simulink model "assembly_crl"  (R2022b)
settings: Solver=FixedStepDiscrete  StartTime=0.0  StopTime=5  RelTol=1e-3  EnableMultiTasking=on
InitFcn:
  | frameSize = 32;
  | numChannels = 2;
  | fs = 44100;
  | maxStages = 4;
  | stagesPerChannel = [1 1];
  | coeffs = [1 0  0 1 0 0; 1 0 0 1 0 0];
  | 
  | firCoeffs = single(zeros(1,32));
  | activeCoeffSet = [0 0];
undefined symbols (not defined in the file or in its folder): carModel, mode
libraries: FeaturePath x1
settings Model: Creator=ap71173  LastModifiedBy=kl13806
settings SolverCC: AlgebraicLoopSolver=TrustRegion
settings OptimizationCC: DefaultParameterBehavior=Inlined  DefaultUnderspecifiedDataType=single  MaxStackSize=2048  EfficientTunableParamExpr=on
settings DebuggingCC: InheritedTsInSrcMsg=none  MultiTaskDSMMsg=none  ParameterPrecisionLossMsg=none  ParameterTunabilityLossMsg=error  UnconnectedInputMsg=warning  UnconnectedOutputMsg=warning  UnconnectedLineMsg=warning  UnknownTsInhSupMsg=none  SFUnexpectedBacktrackingDiag=warning  SFNoUnconditionalDefaultTransitionDiag=warning  SFExecutionAtInitializationDiag=none  SFMachineParentedDataDiag=warning  ArithmeticOperatorsInVariantConditions=warning
settings HardwareCC: ProdBitPerPointer=32  ProdBitPerSizeT=32  ProdBitPerPtrDiffT=32  ProdLargestAtomicInteger=Long  ProdLargestAtomicFloat=Double  ProdEndianess=BigEndian  ProdWordSize=32  ProdHWDeviceType=Custom Processor->Custom  TargetBitPerPointer=64  TargetBitPerSizeT=64  TargetBitPerPtrDiffT=64  TargetLongLongMode=on  TargetIntDivRoundTo=Zero  TargetEndianess=LittleEndian  TargetWordSize=64  TargetHWDeviceType=MATLAB Host
settings ModelReferenceCC: EnableRefExpFcnMdlSchedulingChecks=on
settings SFSimCC: SimUseLocalCustomCode=off  MATLABDynamicMemAlloc=off  CustomCodeUndefinedFunction=UseInterfaceOnly
settings RTWCC: Description=Embedded Coder (host-based shared library target)  SystemTargetFile=ert_shrlib.tlc  TemplateMakefile=ert_default_tmf  GenerateReport=on  RetainRTWFile=on  RTWUseLocalCustomCode=off  Toolchain=ADSP-SC58x v2.3 | gmake makefile (64-bit Windows)  BuildConfiguration=Release - ADSP-SC584  IncludeHyperlinkInReport=on  LaunchReport=on  GenerateTraceInfo=on  GenerateTraceReport=on  GenerateTraceReportSl=on  GenerateTraceReportSf=on  GenerateTraceReportEml=on  GenerateCodeMetricsReport=on  GenerateCodeReplacementReport=on  DLArmComputeVersion=19.05
settings CodeAppCC: ForceParamTrailComments=on  IgnoreCustomStorageClasses=off  OperatorAnnotations=on  SimulinkDataObjDesc=on  SFDataObjDesc=on  MATLABFcnDesc=on  InsertBlockDesc=on  StateflowObjectComments=on  MATLABSourceComments=on
settings STFCustomTargetCC: TargetLangStandard=C99 (ISO)  CodeReplacementLibrary=SHARC+ code replacement libarary  MultiwordLength=256  ParMdlRefBuildCompliant=on  CompOptLevelCompliant=on  CombineOutputUpdateFcns=on  ERTCustomFileBanners=on  SupportContinuousTime=off  SupportNonInlinedSFcns=off  RemoveResetFunc=on  SupportVariableSizeSignals=on  MATLABClassNameForMDSCustomization=Simulink.SoftwareTarget.ERTCustomization  ModelStepFunctionPrototypeControlCompliant=on  UseToolchainInfoCompliant=on  SystemTargetFile=ert_shrlib.tlc
settings ERTTargetCC: TargetLangStandard=C99 (ISO)  CodeReplacementLibrary=SHARC+ code replacement libarary  ConcurrentExecutionCompliant=off  SupportVariableSizeSignals=on  CPPClassGenCompliant=off  InlinedParameterPlacement=NonHierarchical  ERTCustomFileTemplate=example_file_process.tlc  IndentStyle=Allman  IndentSize=4

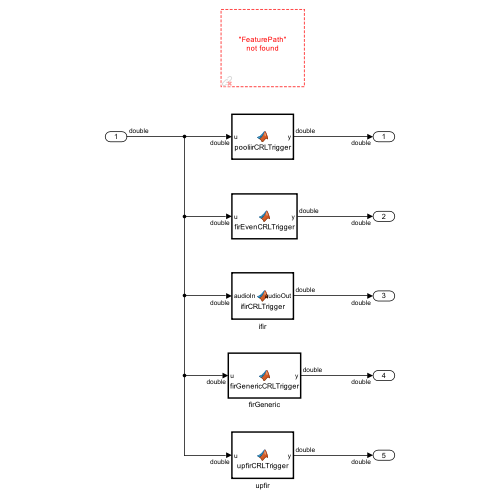
[thumbnail: Simulink's stored preview of the top-level diagram]
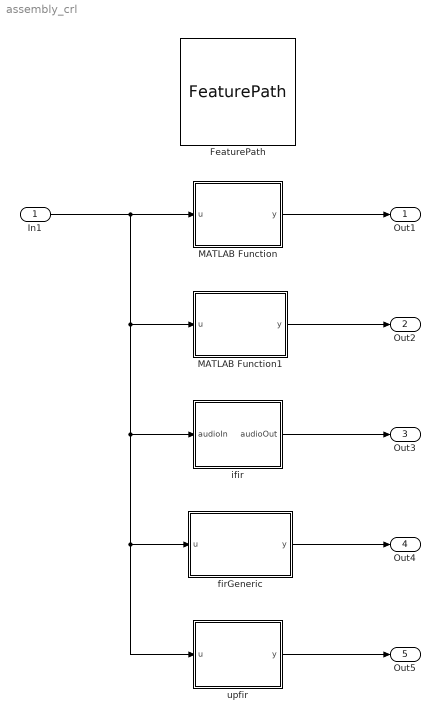
== system assembly_crl ==
  In1 : Inport  OutDataTypeStr=single  PortDimensions=[frameSize numChannels]  SampleTime=frameSize / fs
  FeaturePath : FeaturePath/FeaturePath  FeatureName=assembly_CRL  IsGroup=on  GroupNumber=-1  DeclarePackages=off  PackageNames=mode,carModel  IsToolGroup=off  TriggerInit=[695 419 810 526]
  MATLAB Function : MATLAB Function  TreatAsAtomicUnit=on
  MATLAB Function1 : MATLAB Function  TreatAsAtomicUnit=on
  firGeneric : MATLAB Function  TreatAsAtomicUnit=on
  ifir : MATLAB Function  TreatAsAtomicUnit=on
  upfir : MATLAB Function  TreatAsAtomicUnit=on
  Out1 : Outport  VectorParamsAs1DForOutWhenUnconnected=off
  Out2 : Outport  Port=2  VectorParamsAs1DForOutWhenUnconnected=off
  Out3 : Outport  Port=3  VectorParamsAs1DForOutWhenUnconnected=off
  Out4 : Outport  Port=4  VectorParamsAs1DForOutWhenUnconnected=off
  Out5 : Outport  Port=5  VectorParamsAs1DForOutWhenUnconnected=off
  wires:
  In1/1 -> ifir/1(audioIn), upfir/1(u), firGeneric/1(u), MATLAB Function1/1(u), MATLAB Function/1(u)
  MATLAB Function/1(y) -> Out1/1
  MATLAB Function1/1(y) -> Out2/1
  ifir/1(audioOut) -> Out3/1
  firGeneric/1(y) -> Out4/1
  upfir/1(y) -> Out5/1

== matlab function assembly_crl/MATLAB Function1 ==
  data: u input; y output
function y = firEvenCRLTrigger(u)

firLength = 64;
flipped_coeffs = single(zeros(1,firLength));


% Extract configuration information from inputs
[taps, ~] = size(flipped_coeffs);
[frame_size, num_channels] = size(u);

% Initialize variables
persistent states;
if isempty(states)
    states = single(zeros(taps + 2, num_channels));
end

persistent state_index;
if isempty(state_index)
    state_index = uint32(0);
end

active_coeff_set = zeros(1,num_channels);

% Set correct data types
filter_length = uint32(taps);
frame_size = uint32(frame_size);
num_channels = uint32(num_channels);
active_coeff_set = uint32(active_coeff_set);

y = firEvenCreateAssemblyLib(u, frame_size, num_channels, states, filter_length, state_index, active_coeff_set, flipped_coeffs);


end

function y = firEvenCreateAssemblyLib(u, frame_size, num_channels, states, filter_length, state_index, active_coeff_set, flipped_coeffs)
coder.replace('-errorifnoreplacement');

y = u;

end

== matlab function assembly_crl/MATLAB Function ==
  data: u input; y output single
function y = pooliirCRLTrigger(u)
% This function is intended to trigger the special pooliir CRL which also
% copies the source file into the code gen directory and builds it

[frame_size, num_channels] = size(u);

% Initialize variables
persistent states;
if isempty(states)
    states = single(zeros(size(u)));
end

numStages = uint32(ones(1,num_channels));
coeffs = single(zeros(size(u)));

frame_size = uint32(frame_size);
num_channels = uint32(num_channels);

y = pooliirCreateAssemblyLib(u, frame_size, num_channels, numStages, coeffs, states);
end

function y = pooliirCreateAssemblyLib(u, frame_size, num_channels, numStages, coeffs, states)
coder.replace('-errorifnoreplacement');

y = u;

end

== matlab function assembly_crl/ifir ==
  data: audioIn input; audioOut output
function audioOut = ifirCRLTrigger(audioIn)

I = int32(2);
coeffsFlip = single(zeros(10,1));
% An interpolated FIR filter is an FIR filter with a sparse set of
% coefficients.  That is, the coefficients contain I-1 zeros between
% each point, so the effective length of  filter is len(input_coeffs) * I  
% The function support multiple channels, with each
% channel sharing the same set of filter coefficients.
% 
% p : coefficient set (non-zero coefficients)
% I : interpolation factor, I-1 zeros are inserted between each coefficient
% 
% NOTES: 
% The legacy IFIR block supported coefficient sets.  Currently
% this only supports one coefficient set. 
% The coefficients are stored flipped in time. The unflipped coeffs are
% passed to block mask, and the flipping is done in mask initialization.

% Initialize variables
[frameSize, numChannels] = size(audioIn);
[filterLength, ~] = size(coeffsFlip);

frameSize   = uint32(frameSize);
numChannels = uint32(numChannels);
filterLength = int32(filterLength);
activeCoeffSet = coder.const(uint32(zeros(1,numChannels)));

% State is a circular buffer that holds previous stateLen samples, 
% where state_index points to the last/oldest sample in the buffer, which 
% during processing will be overwritten by the current input sample.
persistent states;
if isempty(states)
    states = single(zeros(20,2));
end

persistent state_index;
if isempty(state_index)
    state_index = int32(0);
end

audioOut = IFIRCreateAssemblyLib(audioIn, frameSize, numChannels, states, filterLength, ...
                    state_index, coeffsFlip, activeCoeffSet, I);
                
end

function y = IFIRCreateAssemblyLib(audioIn, frameSize, numChannels, states2, filterLength, ...
                    state_index2, coeffsFlip, activeCoeffSet, I)
% If code gen'ing, error out if this is not replaced with IFIR.asm
coder.replace('-errorifnoreplacement');

y = audioIn;

end

== matlab function assembly_crl/firGeneric ==
  data: u input; y output
function y = firGenericCRLTrigger(u)
% Generic FIR function to work with M inputs, N outputs and K filters
%
% Parameters:
%   u:              input channels [frame size x number of inputs]
%   coeffs:         coefficient sets [total filter lengths x 1]
%   filterLengths:  array of filter lengths [number of filters x 1]
%   inputMapping:   zero-based input mapping for each filter  [number of outputs x 1]
%   filterMapping:  zero-based filter mapping for each filter [number of outputs x 1]
%
% Global parameters:
%   states:         array of states [totalBufferSize x 1]
%   codeWorkMemory: working memory set up during roommode reset/init CRL
%                   function call [codeWorkMemorySize x 1]

% Extract configuration information from inputs
[frame_size, ~]  = size(u);
num_outputs = 1;

persistent codeWorkMemory;
if isempty(codeWorkMemory)
    codeWorkMemory = uint32(zeros(1,20));
end
    
% Set correct data types
frame_size = uint32(frame_size);
num_outputs = uint32(num_outputs);

y = firGenericCreateAssemblyLib(u, codeWorkMemory, num_outputs);

end

%% CRL functions for code generation
function y = firGenericCreateAssemblyLib(u, workMemory, numOutputs)
% If target == codegen, error out if no CRL found
coder.replace('-errorifnoreplacement');
[frameSize, ~]  = size(u);
y = single(zeros(frameSize, numOutputs));
end

== matlab function assembly_crl/upfir ==
  data: u input; y output
function y = upfirCRLTrigger(u)

firLength = 64;
interp_factor = 4;
flipped_coeffs = single(zeros(1,firLength));

[frame_size, num_channels] = size(u);
[taps, ~] = size(flipped_coeffs);
polyLen = taps/interp_factor;
active_coeff_set = zeros(1,num_channels);

persistent states;
if isempty(states)
    states = single(zeros(taps + 2, num_channels));
end

persistent state_index;
if isempty(state_index)
    state_index = int32(0);
end
filter_length = int32(taps);
frame_size = uint32(frame_size);
num_channels = uint32(num_channels);
active_coeff_set = uint32(active_coeff_set);
interpolation_factor = int32(interp_factor);
polyLen = int32(polyLen);

% isa(u, 'single')
% isa(frame_size, 'uint32')
% isa(num_channels, 'uint32')
% isa(states, 'single')
% isa(filter_length, 'uint32')! int32
% isa(state_index, 'uint32')! int32
% isa(flipped_coeffs, 'single')
% isa(active_coeff_set, 'uint32')
% isa(interpolation_factor, 'int32')
% isa(polyLen, 'int32')


y = upfirCreateAssemblyLib(u, frame_size, num_channels, states, filter_length, state_index, flipped_coeffs, active_coeff_set, interpolation_factor, polyLen);
end

function y = upfirCreateAssemblyLib(u, framesize, numChannels, states2, filterLength, stateIndex2, coeffs, activeCoeffSet, interp_factor, polylen)
coder.replace('-errorifnoreplacement');

y=u;

end
